simulink library "gm_SimplePulseGenerator_4x4_HDL_IQ_lib"  (R2019b)
settings: Solver=VariableStepAuto  StartTime=0.0  StopTime=10.0  RelTol=1e-3
undefined symbols (not defined in the file or in its folder): AXI4, Lite
libraries: axiinterfacelib x16
settings Model: Creator=larry  LastModifiedBy=larry

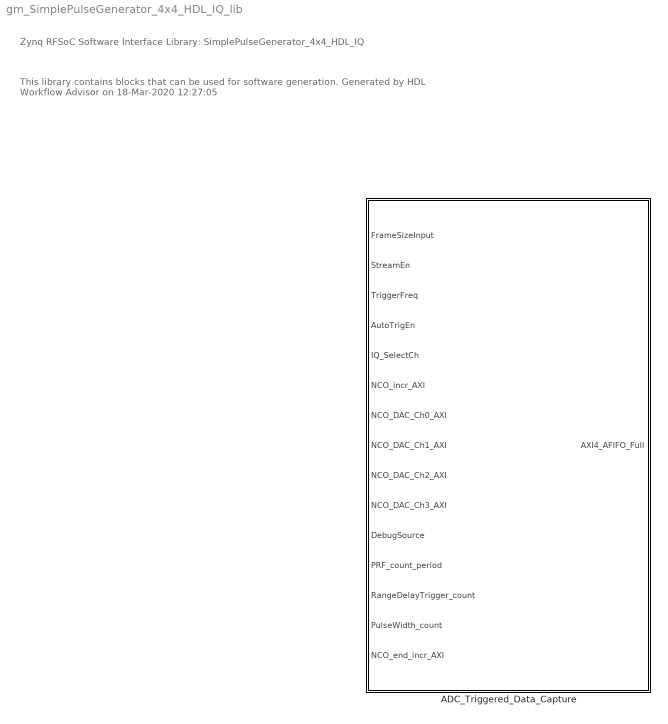
== system gm_SimplePulseGenerator_4x4_HDL_IQ_lib ==
  note: Zynq RFSoC Software Interface Library: SimplePulseGenerator_4x4_HDL_IQ
  note: This library contains blocks that can be used for software generation.
      |
      | Generated by HDL Workflow Advisor on 18-Mar-2020 12:27:05
  ADC_Triggered_Data_Capture : Subsystem  TreatAsAtomicUnit=on  mask(AXI4-Lite/AXI4 Interface){}
      mask help:
      | This is an automatically generated subsystem block.
      | This contains the AXI interface blocks that communicate with the ADC_DAC_IQ_IP IPCore generated from SimplePulseGenerator_4x4_HDL_IQ/ADC_Triggered_Data_Capture subsystem.
      mask Display: disp(sprintf('Xilinx Zynq \nAXI Interface'));

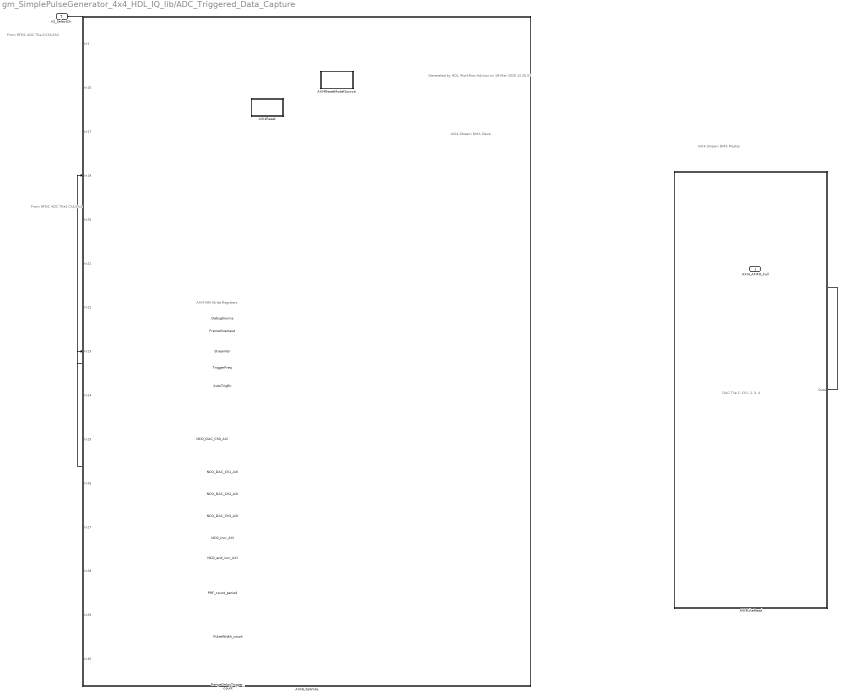
== system gm_SimplePulseGenerator_4x4_HDL_IQ_lib/ADC_Triggered_Data_Capture ==
  note: Generated by HDL Workflow Advisor on 18-Mar-2020 12:26:57
  note: From RFDC ADC Tile1 Ch1/Ch2
  note: DAC Tile 1: Ch1, 2, 3, 4
  note: AXI4-Stream DMA Slave
  note: AXI4-Stream DMA Master
  note: AXI4 MM Write Registers
  note: From RFDC ADC Tile 0 Ch1/Ch2
  FrameSizeInput : Inport
  StreamEn : Inport  Port=2
  TriggerFreq : Inport  Port=3
  AutoTrigEn : Inport  Port=4
  IQ_SelectCh : Inport  Port=5
  NCO_incr_AXI : Inport  Port=6
  NCO_DAC_Ch0_AXI : Inport  Port=7
  NCO_DAC_Ch1_AXI : Inport  Port=8
  NCO_DAC_Ch2_AXI : Inport  Port=9
  NCO_DAC_Ch3_AXI : Inport  Port=10
  DebugSource : Inport  Port=11
  PRF_count_period : Inport  Port=12
  RangeDelayTrigger_count : Inport  Port=13
  PulseWidth_count : Inport  Port=14
  NCO_end_incr_AXI : Inport  Port=15
  AXI4LiteRead : Subsystem  Priority=10
  AXI4LiteWrite : Subsystem  Priority=1
  AXI4Reset : Subsystem  mask(System Start){ShowInLibBrowser=0}
      mask prompts: ShowInLibBrowser "Simulink:masks:CustCodeMaskParam1_MP"
      settings: CopyFcn=cccopyfcn(gcb)  OpenFcn=ccopenfcn('System Start Function')
      mask Help: eval('feval(''rtwprivate'',''rtwhelpview'',''rtw_sys_start_block'')');
      mask Display: disp('System\nStart');
  AXI4ResetModelSource : Subsystem  mask(Model Source){ShowInLibBrowser=0}
      mask prompts: ShowInLibBrowser "Simulink:masks:CustCodeMaskParam1_MP"
      settings: CopyFcn=cccopyfcn(gcb)  OpenFcn=ccopenfcn('Model Source')
      mask Help: eval('feval(''rtwprivate'',''rtwhelpview'',''rtw_model_source_block'')');
      mask Display: disp('Model\nSource');
  AXI4_AFIFO_Full : Outport  VectorParamsAs1DForOutWhenUnconnected=off
  wires:
  AXI4LiteRead/1(Out4) -> AXI4_AFIFO_Full/1
  RangeDelayTrigger_count/1 -> AXI4LiteWrite/15(In30)
  PulseWidth_count/1 -> AXI4LiteWrite/14(In29)
  PRF_count_period/1 -> AXI4LiteWrite/13(In28)
  NCO_end_incr_AXI/1 -> AXI4LiteWrite/12(In27)
  NCO_incr_AXI/1 -> AXI4LiteWrite/11(In26)
  NCO_DAC_Ch3_AXI/1 -> AXI4LiteWrite/10(In25)
  NCO_DAC_Ch2_AXI/1 -> AXI4LiteWrite/9(In24)
  NCO_DAC_Ch1_AXI/1 -> AXI4LiteWrite/8(In23)
  NCO_DAC_Ch0_AXI/1 -> AXI4LiteWrite/7(In22)
  AutoTrigEn/1 -> AXI4LiteWrite/6(In21)
  TriggerFreq/1 -> AXI4LiteWrite/5(In20)
  StreamEn/1 -> AXI4LiteWrite/4(In19)
  FrameSizeInput/1 -> AXI4LiteWrite/3(In17)
  DebugSource/1 -> AXI4LiteWrite/2(In15)
  IQ_SelectCh/1 -> AXI4LiteWrite/1(In1)

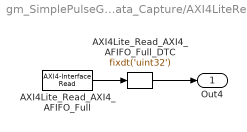
== system gm_SimplePulseGenerator_4x4_HDL_IQ_lib/ADC_Triggered_Data_Capture/AXI4LiteRead ==
  AXI4Lite_Read_AXI4_AFIFO_Full : axiinterfacelib/AXI4-Interface Read  Priority=17  AXIInterfaceType=AXI4-Lite  DeviceName=/dev/mwipcore  RegisterOffset=hex2dec('134')  DataLength=1  DataType=uint32  SampleTime=-1  blockPlatform=ZYNQ  SimulateUsing=Interpreted Execution
      settings: SourceProductName=Embedded Coder Support Package for Xilinx Zynq Platform  SourceProductBaseCode=ECZYNQ7000
  AXI4Lite_Read_AXI4_AFIFO_Full_DTC : DataTypeConversion  OutDataTypeStr=fixdt('uint32')  ConvertRealWorld=Stored Integer (SI)
  Out4 : Outport
  wires:
  AXI4Lite_Read_AXI4_AFIFO_Full_DTC/1 -> Out4/1
  AXI4Lite_Read_AXI4_AFIFO_Full/1 -> AXI4Lite_Read_AXI4_AFIFO_Full_DTC/1

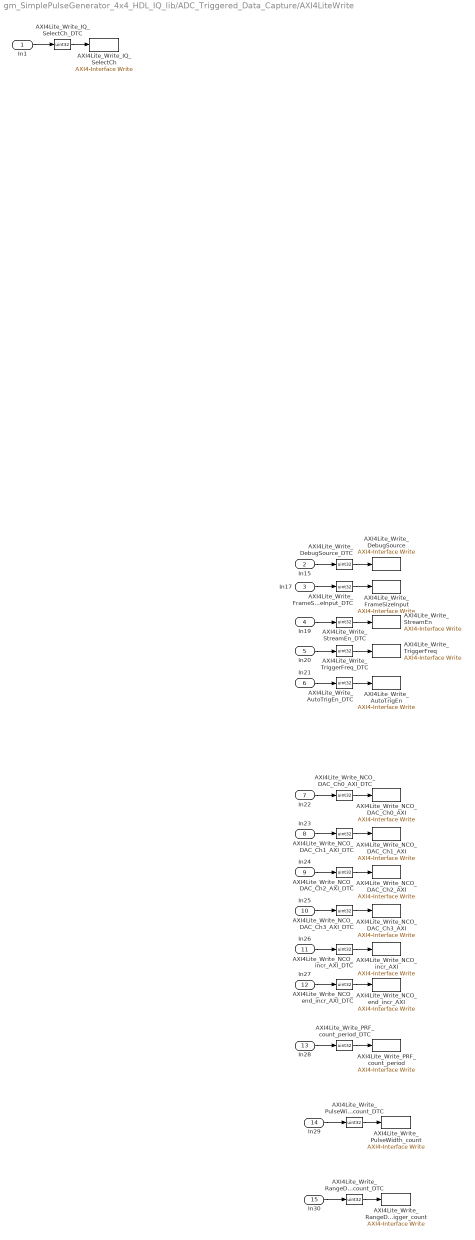
== system gm_SimplePulseGenerator_4x4_HDL_IQ_lib/ADC_Triggered_Data_Capture/AXI4LiteWrite ==
  In1 : Inport
  In15 : Inport  Port=2
  In17 : Inport  Port=3
  In19 : Inport  Port=4
  In20 : Inport  Port=5
  In21 : Inport  Port=6
  In22 : Inport  Port=7
  In23 : Inport  Port=8
  In24 : Inport  Port=9
  In25 : Inport  Port=10
  In26 : Inport  Port=11
  In27 : Inport  Port=12
  In28 : Inport  Port=13
  In29 : Inport  Port=14
  In30 : Inport  Port=15
  AXI4Lite_Write_AutoTrigEn : axiinterfacelib/AXI4-Interface Write  Priority=19  AXIInterfaceType=AXI4-Lite  DeviceName=/dev/mwipcore  RegisterOffset=hex2dec('110')  blockPlatform=ZYNQ  SimulateUsing=Interpreted execution
      settings: SourceProductName=Embedded Coder Support Package for Xilinx Zynq Platform  SourceProductBaseCode=ECZYNQ7000
  AXI4Lite_Write_AutoTrigEn_DTC : DataTypeConversion  OutDataTypeStr=uint32  ConvertRealWorld=Stored Integer (SI)
  AXI4Lite_Write_DebugSource : axiinterfacelib/AXI4-Interface Write  Priority=26  AXIInterfaceType=AXI4-Lite  DeviceName=/dev/mwipcore  RegisterOffset=hex2dec('12C')  blockPlatform=ZYNQ  SimulateUsing=Interpreted execution
      settings: SourceProductName=Embedded Coder Support Package for Xilinx Zynq Platform  SourceProductBaseCode=ECZYNQ7000
  AXI4Lite_Write_DebugSource_DTC : DataTypeConversion  OutDataTypeStr=uint32  ConvertRealWorld=Stored Integer (SI)
  AXI4Lite_Write_FrameSizeInput : axiinterfacelib/AXI4-Interface Write  Priority=16  AXIInterfaceType=AXI4-Lite  DeviceName=/dev/mwipcore  RegisterOffset=hex2dec('104')  blockPlatform=ZYNQ  SimulateUsing=Interpreted execution
      settings: SourceProductName=Embedded Coder Support Package for Xilinx Zynq Platform  SourceProductBaseCode=ECZYNQ7000
  AXI4Lite_Write_FrameSizeInput_DTC : DataTypeConversion  OutDataTypeStr=uint32  ConvertRealWorld=Stored Integer (SI)
  AXI4Lite_Write_IQ_SelectCh : axiinterfacelib/AXI4-Interface Write  Priority=20  AXIInterfaceType=AXI4-Lite  DeviceName=/dev/mwipcore  RegisterOffset=hex2dec('114')  blockPlatform=ZYNQ  SimulateUsing=Interpreted execution
      settings: SourceProductName=Embedded Coder Support Package for Xilinx Zynq Platform  SourceProductBaseCode=ECZYNQ7000
  AXI4Lite_Write_IQ_SelectCh_DTC : DataTypeConversion  OutDataTypeStr=uint32  ConvertRealWorld=Stored Integer (SI)
  AXI4Lite_Write_NCO_DAC_Ch0_AXI : axiinterfacelib/AXI4-Interface Write  Priority=22  AXIInterfaceType=AXI4-Lite  DeviceName=/dev/mwipcore  RegisterOffset=hex2dec('11C')  blockPlatform=ZYNQ  SimulateUsing=Interpreted execution
      settings: SourceProductName=Embedded Coder Support Package for Xilinx Zynq Platform  SourceProductBaseCode=ECZYNQ7000
  AXI4Lite_Write_NCO_DAC_Ch0_AXI_DTC : DataTypeConversion  OutDataTypeStr=uint32  ConvertRealWorld=Stored Integer (SI)
  AXI4Lite_Write_NCO_DAC_Ch1_AXI : axiinterfacelib/AXI4-Interface Write  Priority=23  AXIInterfaceType=AXI4-Lite  DeviceName=/dev/mwipcore  RegisterOffset=hex2dec('120')  blockPlatform=ZYNQ  SimulateUsing=Interpreted execution
      settings: SourceProductName=Embedded Coder Support Package for Xilinx Zynq Platform  SourceProductBaseCode=ECZYNQ7000
  AXI4Lite_Write_NCO_DAC_Ch1_AXI_DTC : DataTypeConversion  OutDataTypeStr=uint32  ConvertRealWorld=Stored Integer (SI)
  AXI4Lite_Write_NCO_DAC_Ch2_AXI : axiinterfacelib/AXI4-Interface Write  Priority=24  AXIInterfaceType=AXI4-Lite  DeviceName=/dev/mwipcore  RegisterOffset=hex2dec('124')  blockPlatform=ZYNQ  SimulateUsing=Interpreted execution
      settings: SourceProductName=Embedded Coder Support Package for Xilinx Zynq Platform  SourceProductBaseCode=ECZYNQ7000
  AXI4Lite_Write_NCO_DAC_Ch2_AXI_DTC : DataTypeConversion  OutDataTypeStr=uint32  ConvertRealWorld=Stored Integer (SI)
  AXI4Lite_Write_NCO_DAC_Ch3_AXI : axiinterfacelib/AXI4-Interface Write  Priority=25  AXIInterfaceType=AXI4-Lite  DeviceName=/dev/mwipcore  RegisterOffset=hex2dec('128')  blockPlatform=ZYNQ  SimulateUsing=Interpreted execution
      settings: SourceProductName=Embedded Coder Support Package for Xilinx Zynq Platform  SourceProductBaseCode=ECZYNQ7000
  AXI4Lite_Write_NCO_DAC_Ch3_AXI_DTC : DataTypeConversion  OutDataTypeStr=uint32  ConvertRealWorld=Stored Integer (SI)
  AXI4Lite_Write_NCO_end_incr_AXI : axiinterfacelib/AXI4-Interface Write  Priority=30  AXIInterfaceType=AXI4-Lite  DeviceName=/dev/mwipcore  RegisterOffset=hex2dec('100')  blockPlatform=ZYNQ  SimulateUsing=Interpreted execution
      settings: SourceProductName=Embedded Coder Support Package for Xilinx Zynq Platform  SourceProductBaseCode=ECZYNQ7000
  AXI4Lite_Write_NCO_end_incr_AXI_DTC : DataTypeConversion  OutDataTypeStr=uint32  ConvertRealWorld=Stored Integer (SI)
  AXI4Lite_Write_NCO_incr_AXI : axiinterfacelib/AXI4-Interface Write  Priority=21  AXIInterfaceType=AXI4-Lite  DeviceName=/dev/mwipcore  RegisterOffset=hex2dec('118')  blockPlatform=ZYNQ  SimulateUsing=Interpreted execution
      settings: SourceProductName=Embedded Coder Support Package for Xilinx Zynq Platform  SourceProductBaseCode=ECZYNQ7000
  AXI4Lite_Write_NCO_incr_AXI_DTC : DataTypeConversion  OutDataTypeStr=uint32  ConvertRealWorld=Stored Integer (SI)
  AXI4Lite_Write_PRF_count_period : axiinterfacelib/AXI4-Interface Write  Priority=27  AXIInterfaceType=AXI4-Lite  DeviceName=/dev/mwipcore  RegisterOffset=hex2dec('130')  blockPlatform=ZYNQ  SimulateUsing=Interpreted execution
      settings: SourceProductName=Embedded Coder Support Package for Xilinx Zynq Platform  SourceProductBaseCode=ECZYNQ7000
  AXI4Lite_Write_PRF_count_period_DTC : DataTypeConversion  OutDataTypeStr=uint32  ConvertRealWorld=Stored Integer (SI)
  AXI4Lite_Write_PulseWidth_count : axiinterfacelib/AXI4-Interface Write  Priority=29  AXIInterfaceType=AXI4-Lite  DeviceName=/dev/mwipcore  RegisterOffset=hex2dec('13C')  blockPlatform=ZYNQ  SimulateUsing=Interpreted execution
      settings: SourceProductName=Embedded Coder Support Package for Xilinx Zynq Platform  SourceProductBaseCode=ECZYNQ7000
  AXI4Lite_Write_PulseWidth_count_DTC : DataTypeConversion  OutDataTypeStr=uint32  ConvertRealWorld=Stored Integer (SI)
  AXI4Lite_Write_RangeDelayTrigger_count : axiinterfacelib/AXI4-Interface Write  Priority=28  AXIInterfaceType=AXI4-Lite  DeviceName=/dev/mwipcore  RegisterOffset=hex2dec('138')  blockPlatform=ZYNQ  SimulateUsing=Interpreted execution
      settings: SourceProductName=Embedded Coder Support Package for Xilinx Zynq Platform  SourceProductBaseCode=ECZYNQ7000
  AXI4Lite_Write_RangeDelayTrigger_count_DTC : DataTypeConversion  OutDataTypeStr=uint32  ConvertRealWorld=Stored Integer (SI)
  AXI4Lite_Write_StreamEn : axiinterfacelib/AXI4-Interface Write  Priority=17  AXIInterfaceType=AXI4-Lite  DeviceName=/dev/mwipcore  RegisterOffset=hex2dec('108')  blockPlatform=ZYNQ  SimulateUsing=Interpreted execution
      settings: SourceProductName=Embedded Coder Support Package for Xilinx Zynq Platform  SourceProductBaseCode=ECZYNQ7000
  AXI4Lite_Write_StreamEn_DTC : DataTypeConversion  OutDataTypeStr=uint32  ConvertRealWorld=Stored Integer (SI)
  AXI4Lite_Write_TriggerFreq : axiinterfacelib/AXI4-Interface Write  Priority=18  AXIInterfaceType=AXI4-Lite  DeviceName=/dev/mwipcore  RegisterOffset=hex2dec('10C')  blockPlatform=ZYNQ  SimulateUsing=Interpreted execution
      settings: SourceProductName=Embedded Coder Support Package for Xilinx Zynq Platform  SourceProductBaseCode=ECZYNQ7000
  AXI4Lite_Write_TriggerFreq_DTC : DataTypeConversion  OutDataTypeStr=uint32  ConvertRealWorld=Stored Integer (SI)
  wires:
  In20/1 -> AXI4Lite_Write_TriggerFreq_DTC/1
  In17/1 -> AXI4Lite_Write_FrameSizeInput_DTC/1
  In28/1 -> AXI4Lite_Write_PRF_count_period_DTC/1
  In1/1 -> AXI4Lite_Write_IQ_SelectCh_DTC/1
  AXI4Lite_Write_NCO_end_incr_AXI_DTC/1 -> AXI4Lite_Write_NCO_end_incr_AXI/1
  In26/1 -> AXI4Lite_Write_NCO_incr_AXI_DTC/1
  AXI4Lite_Write_TriggerFreq_DTC/1 -> AXI4Lite_Write_TriggerFreq/1
  AXI4Lite_Write_IQ_SelectCh_DTC/1 -> AXI4Lite_Write_IQ_SelectCh/1
  AXI4Lite_Write_StreamEn_DTC/1 -> AXI4Lite_Write_StreamEn/1
  In29/1 -> AXI4Lite_Write_PulseWidth_count_DTC/1
  In15/1 -> AXI4Lite_Write_DebugSource_DTC/1
  AXI4Lite_Write_NCO_DAC_Ch1_AXI_DTC/1 -> AXI4Lite_Write_NCO_DAC_Ch1_AXI/1
  AXI4Lite_Write_DebugSource_DTC/1 -> AXI4Lite_Write_DebugSource/1
  AXI4Lite_Write_PulseWidth_count_DTC/1 -> AXI4Lite_Write_PulseWidth_count/1
  In19/1 -> AXI4Lite_Write_StreamEn_DTC/1
  AXI4Lite_Write_NCO_incr_AXI_DTC/1 -> AXI4Lite_Write_NCO_incr_AXI/1
  AXI4Lite_Write_PRF_count_period_DTC/1 -> AXI4Lite_Write_PRF_count_period/1
  In24/1 -> AXI4Lite_Write_NCO_DAC_Ch2_AXI_DTC/1
  In22/1 -> AXI4Lite_Write_NCO_DAC_Ch0_AXI_DTC/1
  In25/1 -> AXI4Lite_Write_NCO_DAC_Ch3_AXI_DTC/1
  AXI4Lite_Write_RangeDelayTrigger_count_DTC/1 -> AXI4Lite_Write_RangeDelayTrigger_count/1
  In30/1 -> AXI4Lite_Write_RangeDelayTrigger_count_DTC/1
  In21/1 -> AXI4Lite_Write_AutoTrigEn_DTC/1
  AXI4Lite_Write_NCO_DAC_Ch2_AXI_DTC/1 -> AXI4Lite_Write_NCO_DAC_Ch2_AXI/1
  AXI4Lite_Write_NCO_DAC_Ch3_AXI_DTC/1 -> AXI4Lite_Write_NCO_DAC_Ch3_AXI/1
  In23/1 -> AXI4Lite_Write_NCO_DAC_Ch1_AXI_DTC/1
  In27/1 -> AXI4Lite_Write_NCO_end_incr_AXI_DTC/1
  AXI4Lite_Write_NCO_DAC_Ch0_AXI_DTC/1 -> AXI4Lite_Write_NCO_DAC_Ch0_AXI/1
  AXI4Lite_Write_FrameSizeInput_DTC/1 -> AXI4Lite_Write_FrameSizeInput/1
  AXI4Lite_Write_AutoTrigEn_DTC/1 -> AXI4Lite_Write_AutoTrigEn/1

== system gm_SimplePulseGenerator_4x4_HDL_IQ_lib/ADC_Triggered_Data_Capture/AXI4Reset ==

== system gm_SimplePulseGenerator_4x4_HDL_IQ_lib/ADC_Triggered_Data_Capture/AXI4ResetModelSource ==
